simulink model "TEST1"  (R2024b)
settings: Solver=ode4  StartTime=0.0  StopTime=100  FixedStep=0.01  RelTol=1e-3
libraries: slpidlib x1, simulink x1
settings Model: LastModifiedBy=Arshaan Parwez

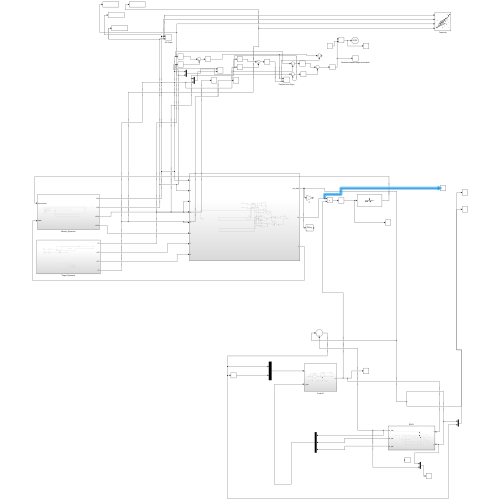
[thumbnail: Simulink's stored preview of the top-level diagram]
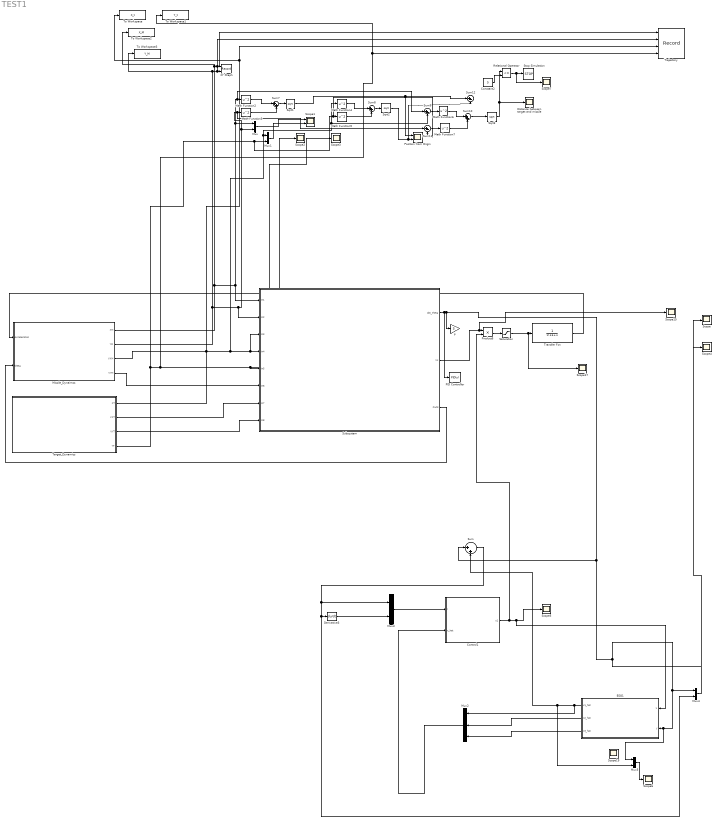
== system TEST1 ==
  Constant2 : Constant  Value=5
  Control1 : Subsystem
  Derivative3 : Derivative
  Distance between target and missile : Scope
  ESO1 : Subsystem
  Math Function{2..7} (6 alike) : Math  Operator=square
  Missile_Dynaimcs : Subsystem
  Mux{,1,3..5} (5 alike) : Mux  Inputs=2
  Mux2 : Mux  Inputs=3
  P : Gain  Gain=3
  PID Controller : slpidlib/PID Controller  Controller=PID  Form=Parallel  TimeDomain=Continuous-time  UseExternalTs=off  SampleTime=-1  IntegratorMethod=Forward Euler  FilterMethod=Forward Euler  ControllerParametersSource=internal  P=3  I=2  UseKiTs=off  D=1.5  UseExternalDerivativeSource=off  N=100  UseFilter=on  TunerSelectOption=Transfer Function Based (PID Tuner App)  InitialConditionSource=internal  InitialConditionForIntegrator=0  InitialConditionForFilter=0  DifferentiatorICPrevScaledInput=0  ExternalReset=none  TrackingMode=off  Kt=1  LimitOutput=off  SatLimitsSource=internal  UpperSaturationLimit=inf  LowerSaturationLimit=-inf  LinearizeAsGain=on  AntiWindupMode=none  Kb=1  LimitIntegrator=off  UpperIntegratorSaturationLimit=inf  LowerIntegratorSaturationLimit=-inf  POutMin=[]  POutMax=[]  IOutMin=[]  IOutMax=[]  DOutMin=[]  DOutMax=[]  NOutMin=[]  NOutMax=[]  SumOutMin=[]  SumOutMax=[]  SaturationOutMin=[]  SaturationOutMax=[]  PParamMin=[]  PParamMax=[]  IParamMin=[]  IParamMax=[]  DParamMin=[]  DParamMax=[]  NParamMin=[]  NParamMax=[]  KbParamMin=[]  KbParamMax=[]  KtParamMin=[]  KtParamMax=[]  KbOutMin=[]  KbOutMax=[]  KtOutMin=[]  KtOutMax=[]  IntegratorOutMin=[]  IntegratorOutMax=[]  FilterOutMin=[]  FilterOutMax=[]  SumI1OutMin=[]  SumI1OutMax=[]  SumI2OutMin=[]  SumI2OutMax=[]  SumI3OutMin=[]  SumI3OutMax=[]  SumI4OutMin=[]  SumI4OutMax=[]  SumDOutMin=[]  SumDOutMax=[]  DifferentiatorOutMin=[]  DifferentiatorOutMax=[]  FilterDiffOutCoefMin=[]  FilterDiffOutCoefMax=[]  ReciprocalOutMin=[]  ReciprocalOutMax=[]  SumDenOutMin=[]  SumDenOutMax=[]  SumNumOutMin=[]  SumNumOutMax=[]  DivideOutMin=[]  DivideOutMax=[]  UdiffTsProdOutMin=[]  UdiffTsProdOutMax=[]  NTsProdOutMin=[]  NTsProdOutMax=[]  UintegralTsProdOutMin=[]  UintegralTsProdOutMax=[]  UngainTsProdOutMin=[]  UngainTsProdOutMax=[]  ClampingZeroOutDataTypeStr=Inherit: Inherit via back propagation  ClampingZeroOutMin=[]  ClampingZeroOutMax=[]  FilterDenConstantOutDataTypeStr=Inherit: Inherit via back propagation  FilterDenConstantOutMin=[]  FilterDenConstantOutMax=[]  PCopyOutDataTypeStr=Inherit: Inherit via back propagation  PCopyOutMin=[]  PCopyOutMax=[]  NCopyOutDataTypeStr=Inherit: Inherit via back propagation  NCopyOutMin=[]  NCopyOutMax=[]  IntegratorContinuousStateAttributes=''  IntegratorStateMustResolveToSignalObject=off  IntegratorRTWStateStorageClass=Auto  FilterContinuousStateAttributes=''  FilterStateMustResolveToSignalObject=off  FilterRTWStateStorageClass=Auto  ParallelPVariant=InternalParameters  IdealPVariant=Disabled  IVariant=InternalParameters  DVariant=InternalParameters  IntegratorVariant=Continuous  SatVariant=Disabled  AWVariant=Passthrough  PCopyVariant=Disabled  TRVariant=Disabled  FdbkBlocksVariant=Forward  IdealPFdbkVariant=Disabled  SatFdbkVariant=Disabled  DerivativeFilterVariant=ContFilter  NVariant=InternalParameters  NCopyVariant=Disabled  FilterICVariant=InternalICsFilter  IntegratorICVariant=InternalICs  ExternalResetVariant=Disabled  TRSumVariant=Passthrough  SumFdbkVariant=Disabled  SumVariant=Sum_PID  TsampFilterVariant=InternalTs  TsampNgainVariant=Passthrough  TsampIntegralVariant=Disabled_SignalSpec  ExternalSaturationOutDataTypeStr=Inherit: Same as second input  DerivativeSourceVariant=ErrorSignal  PreIntVariant=InternalPreInt
  Position from Origin : Scope  NumInputPorts=2
  Product6 : Product
  Relational Operator : RelationalOperator  Operator=<=  OutDataTypeStr=boolean  RndMeth=Simplest  InputSameDT=off
  Saturation : Saturate  UpperLimit=50  LowerLimit=-50
  Scope{,2..7,15,17,19} (10 alike) : Scope
  Scope1 : Scope  NumInputPorts=2
  Sqrt1 : Sqrt
  Sqrt2 : Sqrt
  Sqrt3 : Sqrt
  Stop Simulation : Stop
  Subsystem : Subsystem
  Sum{,7..8,10} (4 alike) : Sum  Inputs=|++
  Sum11 : Sum  Inputs=|+-
  Sum12 : Sum  Inputs=|+-
  Sum9 : Sum  Inputs=|+-
  Target_Dynamics : Subsystem
  To Workspace : ToWorkspace  VariableName=X_t  SaveFormat=Timeseries  SampleTime=-1
  To Workspace1 : ToWorkspace  VariableName=Y_t  SaveFormat=Timeseries  SampleTime=-1
  To Workspace2 : ToWorkspace  VariableName=X_M  SaveFormat=Timeseries  SampleTime=-1
  To Workspace3 : ToWorkspace  VariableName=Y_M  SaveFormat=Timeseries  SampleTime=-1
  Trajectory : Record  FileSettingsInternal="{\"entries\":[{\"content\":{\"excelSettings\":{\"content\":{},\"type\":\"Streamout.ExcelSettings\"}},\"type\":\"Streamout.FileSettingStorage\",\"uuid\":\"\"}],\"packageUris\":[\"http:\\/\\/schema.mathworks.com\\/mf0\\/streamout_blocks\\/R2020a\"],\"version\":\"1.0\"}"  Layout=[1 1]  SignalsInternal="{\"entries\":[{\"content\":{\"signals\":[{\"content\":{\"blockPath\":[],\"dimensions\":[1],\"domain\":\"\",\"lineColor\":\"#fe330a\",\"lineWidth\":2,\"plots\":[ 1 ],\"port\":1,\"sid\":[\"\"],\"signalID\":1,\"signalName\":\"Missile_Dynaimcs:1\"},\"type\":\"RecordBlkView.Signal\",\"uuid\":\"\"},{\"content\":{\"blockPath\":[],\"dimensions\":[1],\"domain\":\"\",\"lineColor\":\"#d95319\",\"lineWidth\":2,\"plots\":[ 1 ],\"port\":2,\"sid\":[\"\"],\"signalID\":2,\"signalName\":\"Missile_Dynaimcs:2\"},\"type\":\"RecordBlkView.Signal\",\"uuid\":\"\"},{\"content\":{\"blockPath\":[],\"dimensions\":[1],\"domain\":\"\",\"lineColor\":\"#0072bd\",\"lineWidth\":2,\"plots\":[ 1 ],\"port\":3,\"sid\":[\"\"],\"signalID\":3,\"signalName\":\"Target_Dynamics:1\"},\"type\":\"RecordBlkView.Signal\",\"uuid\":\"\"},{\"content\":{\"blockPath\":[],\"dimensions\":[1],\"domain\":\"\",\"lineColor\":\"#0072bd\",\"lineWidth\":2,\"plots\":[ 1 ],\"port\":4,\"sid\":[\"\"],\"signalID\":4,\"signalName\":\"Target_Dynamics:4\"},\"type\":\"RecordBlkView.Signal\",\"uuid\":\"\"}]},\"type\":\"RecordBlkView.InputSignals\",\"uuid\":\"\"}],\"packageUris\":[\"http:\\/\\/schema.mathworks.com\\/mf0\\/streamout_blocks\\/R2020a\"],\"version\":\"1.0\"}"  VisualizationBindings="{\"xyplotplugin\":{\"info\":[{\"series\":[{\"bindingParametersList\":[{\"parameter\":\"X-Axis\",\"signalID\":1,\"signalName\":\"Missile_Dynaimcs:1\"},{\"parameter\":\"Y-Axis\",\"signalID\":2,\"signalName\":\"Missile_Dynaimcs:2\"}],\"seriesID\":0},{\"bindingParametersList\":[{\"parameter\":\"X-Axis\",\"signalID\":3,\"signalName\":\"Target_Dynamics:1\"},{\"parameter\":\"Y-Axis\",\"signalID\":4,\"signalName\":\"Target_Dynamics:4\"}],\"seriesID\":1}],\"subplotID\":1}]}}"  CompatibilityTag=XY
  Transfer Fcn : TransferFcn  Denominator=[0.1 1]
  XY Graph : Record  FileSettingsInternal="{\"entries\":[{\"content\":{\"excelSettings\":{\"content\":{},\"type\":\"Streamout.ExcelSettings\"}},\"type\":\"Streamout.FileSettingStorage\",\"uuid\":\"\"}],\"packageUris\":[\"http:\\/\\/schema.mathworks.com\\/mf0\\/streamout_blocks\\/R2020a\"],\"version\":\"1.0\"}"  Layout=[1 1]  SignalsInternal="{\"entries\":[{\"content\":{\"signals\":[{\"content\":{\"blockPath\":[],\"dimensions\":[1],\"domain\":\"\",\"lineColor\":\"#64d413\",\"lineWidth\":2,\"port\":1,\"sid\":[\"\"],\"signalID\":1,\"signalName\":\"Missile_Dynaimcs:1\"},\"type\":\"RecordBlkView.Signal\",\"uuid\":\"\"},{\"content\":{\"blockPath\":[],\"dimensions\":[1],\"domain\":\"\",\"lineColor\":\"#ff13a6\",\"lineWidth\":2,\"port\":2,\"sid\":[\"\"],\"signalID\":2,\"signalName\":\"Missile_Dynaimcs:2\"},\"type\":\"RecordBlkView.Signal\",\"uuid\":\"\"}]},\"type\":\"RecordBlkView.InputSignals\",\"uuid\":\"\"}],\"packageUris\":[\"http:\\/\\/schema.mathworks.com\\/mf0\\/streamout_blocks\\/R2020a\"],\"version\":\"1.0\"}"  VisualizationBindings="{\"xyplotplugin\":{\"info\":[{\"series\":[],\"subplotID\":1}]}}"  CompatibilityTag=XY
  wires:
  Transfer Fcn/1 -> Missile_Dynaimcs/1(Acceleration)
  Mux/1 -> Scope1/1
  Mux1/1 -> Scope1/2
  Math Function2/1 -> Sum7/1
  Math Function3/1 -> Sum7/2
  Sum7/1 -> Sqrt1/1
  Math Function4/1 -> Sum8/1
  Sum8/1 -> Sqrt2/1
  Math Function5/1 -> Sum8/2
  Sqrt1/1 -> Sum12/1, Position from Origin/1
  Sqrt2/1 -> Sum12/2, Position from Origin/2
  Relational Operator/1 -> Scope7/1, Stop Simulation/1
  Sum9/1 -> Math Function6/1
  Sum11/1 -> Math Function7/1
  Math Function6/1 -> Sum10/1
  Math Function7/1 -> Sum10/2
  Sum10/1 -> Sqrt3/1
  Constant2/1 -> Relational Operator/2
  Target_Dynamics/1(XT) -> To Workspace/1, Trajectory/3, Math Function4/1, Sum9/2, Mux1/1, Scope2/1, Subsystem/3(In3)
  Target_Dynamics/4(YT) -> Sum11/2, Math Function5/1, Mux1/2, To Workspace1/1, Trajectory/4, Scope3/1, Subsystem/5(In5)
  Missile_Dynaimcs/1(XM) -> To Workspace2/1, Trajectory/1, XY Graph/1, Subsystem/1(In1), Sum9/1, Math Function2/1, Mux/1
  Missile_Dynaimcs/2(YM) -> To Workspace3/1, Trajectory/2, XY Graph/2, Subsystem/2(In2), Sum11/1, Math Function3/1, Mux/2
  Missile_Dynaimcs/3(VXM) -> Subsystem/4(In4)
  Missile_Dynaimcs/4(VYM) -> Subsystem/6(In6)
  Target_Dynamics/2(VXT) -> Subsystem/7(In7)
  Target_Dynamics/3(VYT) -> Subsystem/8(In8)
  Subsystem/3(Out3) -> Missile_Dynaimcs/2(theta)
  Sqrt3/1 -> Distance between target and missile/1, Relational Operator/1
  Derivative3/1 -> Mux3/2
  Mux3/1 -> Control1/1(r)
  Sum/1 -> Mux4/2, Derivative3/1, Mux3/1
  ESO1/1(x1_hat) -> Mux2/1, Sum/2, Mux5/2
  Mux2/1 -> Control1/2(x_hat)
  Mux4/1 -> Scope4/1
  Mux5/1 -> Scope6/1
  Subsystem/1(dot_theta) -> PID Controller/1, P/1, Sum/1, Mux4/1, ESO1/2(y), Mux5/1, Scope/1
  Control1/1(u1) -> Product6/2, ESO1/1(u), Scope5/1
  Subsystem/2(Vc) -> Scope15/1, Product6/1
  ESO1/2(x2_hat) -> Mux2/2
  ESO1/3(x3_hat) -> Mux2/3
  Product6/1 -> Saturation/1
  Saturation/1 -> Scope17/1, Transfer Fcn/1

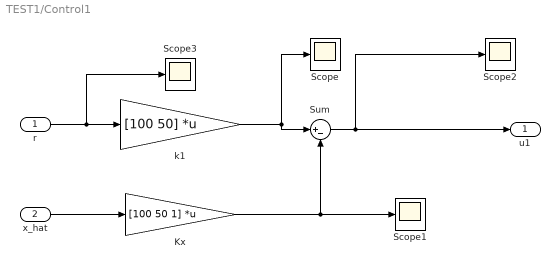
== system TEST1/Control1 ==
  r : Inport
  x_hat : Inport  Port=2
  Kx : Gain  Gain=[100 50 1]  Multiplication=Matrix(K*u)
  Scope{,1..3} (4 alike) : Scope
  Sum : Sum  Inputs=|+-
  k1 : Gain  Gain=[100 50]  Multiplication=Matrix(K*u)
  u1 : Outport
  wires:
  Sum/1 -> u1/1, Scope2/1
  Kx/1 -> Scope1/1, Sum/2
  k1/1 -> Sum/1, Scope/1
  x_hat/1 -> Kx/1
  r/1 -> Scope3/1, k1/1

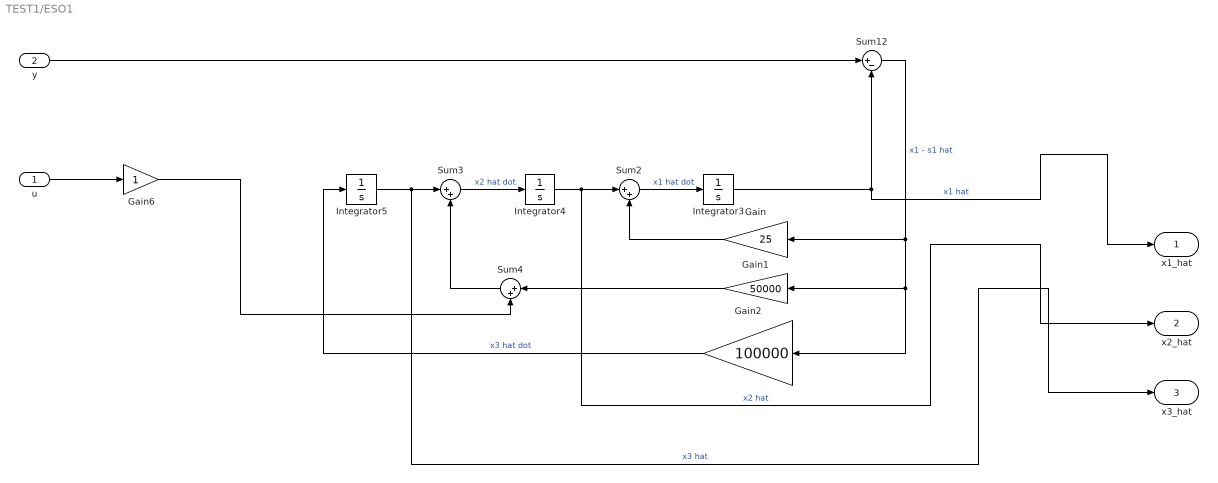
== system TEST1/ESO1 ==
  u : Inport
  y : Inport  Port=2
  Gain : Gain  Gain=25
  Gain1 : Gain  Gain=50000
  Gain2 : Gain  Gain=100000
  Gain6 : Gain
  Integrator3 : Integrator
  Integrator4 : Integrator
  Integrator5 : Integrator
  Sum12 : Sum  Inputs=|+-
  Sum2 : Sum  Inputs=|++
  Sum3 : Sum  Inputs=|++
  Sum4 : Sum  Inputs=|++
  x1_hat : Outport
  x2_hat : Outport  Port=2
  x3_hat : Outport  Port=3
  wires:
  Gain1/1 -> Sum4/1
  Sum12/1 -> Gain/1, Gain1/1, Gain2/1  "x1 - s1 hat"
  Sum4/1 -> Sum3/2
  Integrator4/1 -> x2_hat/1, Sum2/1  "x2 hat"
  Integrator3/1 -> x1_hat/1, Sum12/2  "x1 hat"
  Gain2/1 -> Integrator5/1  "x3 hat dot"
  y/1 -> Sum12/1
  u/1 -> Gain6/1
  Sum3/1 -> Integrator4/1  "x2 hat dot"
  Gain6/1 -> Sum4/2
  Gain/1 -> Sum2/2
  Integrator5/1 -> Sum3/1, x3_hat/1  "x3 hat"
  Sum2/1 -> Integrator3/1  "x1 hat dot"

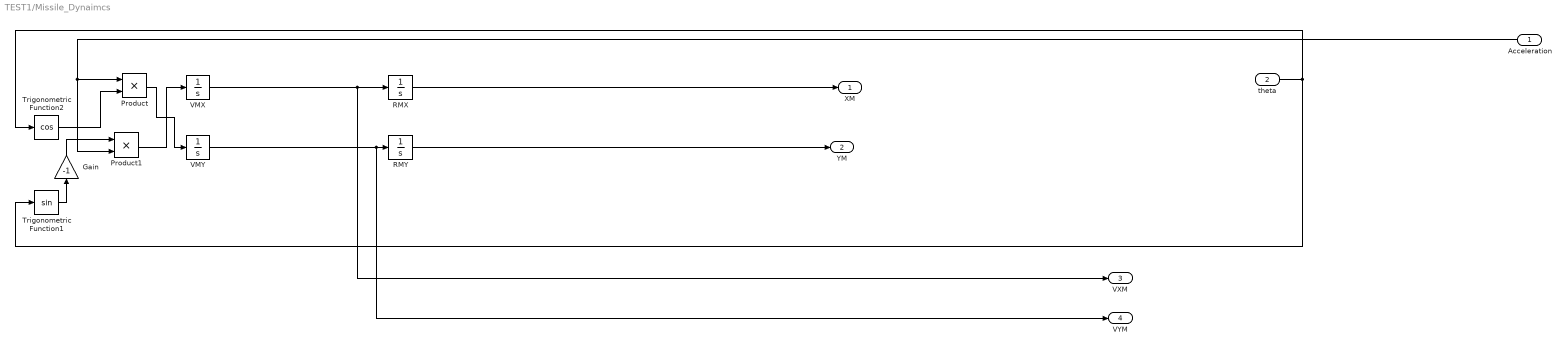
== system TEST1/Missile_Dynaimcs ==
  Acceleration : Inport
  theta : Inport  Port=2
  Gain : Gain  Gain=-1
  Product : Product
  Product1 : Product
  RMX : Integrator
  RMY : Integrator  InitialCondition=3000
  Trigonometric Function1 : Trigonometry
  Trigonometric Function2 : Trigonometry  Operator=cos
  VMX : Integrator  InitialCondition=600
  VMY : Integrator  InitialCondition=100
  XM : Outport
  YM : Outport  Port=2
  VXM : Outport  Port=3
  VYM : Outport  Port=4
  wires:
  Trigonometric Function1/1 -> Gain/1
  VMX/1 -> VXM/1, RMX/1
  theta/1 -> Trigonometric Function1/1, Trigonometric Function2/1
  Trigonometric Function2/1 -> Product/2
  RMX/1 -> XM/1
  Acceleration/1 -> Product1/2, Product/1
  Product/1 -> VMY/1
  Product1/1 -> VMX/1
  VMY/1 -> VYM/1, RMY/1
  Gain/1 -> Product1/1
  RMY/1 -> YM/1

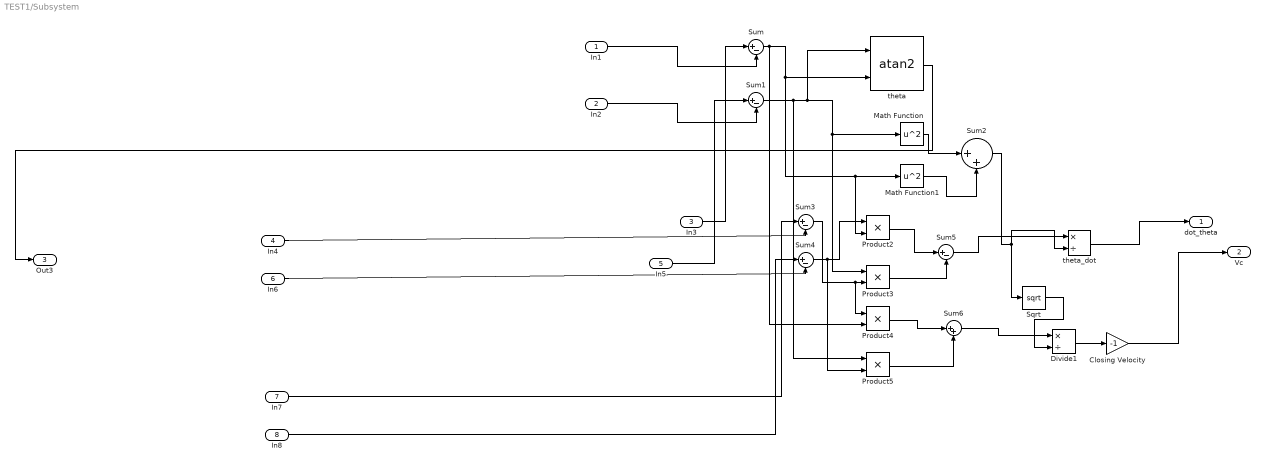
== system TEST1/Subsystem ==
  In1 : Inport
  In2 : Inport  Port=2
  In3 : Inport  Port=3
  In4 : Inport  Port=4
  In5 : Inport  Port=5
  In6 : Inport  Port=6
  In7 : Inport  Port=7
  In8 : Inport  Port=8
  Closing Velocity : Gain  Gain=-1
  Divide1 : Product  Inputs=*/
  Math Function : Math  Operator=square
  Math Function1 : Math  Operator=square
  Product{2..5} (4 alike) : Product
  Sqrt : Sqrt
  Sum{,1,3..5} (5 alike) : Sum  Inputs=|+-
  Sum2 : Sum  Inputs=|++
  Sum6 : Sum  Inputs=|++
  theta : Trigonometry  Operator=atan2
  theta_dot : Product  Inputs=*/
  dot_theta : Outport
  Vc : Outport  Port=2
  Out3 : Outport  Port=3
  wires:
  Math Function/1 -> Sum2/1
  Sum2/1 -> Sqrt/1, theta_dot/2
  Sum3/1 -> Product4/1, Product3/2
  Sum/1 -> Product4/2, Product2/2, Math Function1/1, theta/2
  Product4/1 -> Sum6/1
  Product2/1 -> Sum5/1
  Sum6/1 -> Divide1/1
  Math Function1/1 -> Sum2/2
  Sum4/1 -> Product5/2, Product2/1
  Sqrt/1 -> Divide1/2
  Divide1/1 -> Closing Velocity/1
  Product5/1 -> Sum6/2
  In3/1 -> Sum/1
  In7/1 -> Sum3/1
  Sum1/1 -> Product5/1, Product3/1, Math Function/1, theta/1
  theta_dot/1 -> dot_theta/1
  In8/1 -> Sum4/1
  In1/1 -> Sum/2
  theta/1 -> Out3/1
  Closing Velocity/1 -> Vc/1
  In5/1 -> Sum1/1
  In4/1 -> Sum3/2
  Product3/1 -> Sum5/2
  Sum5/1 -> theta_dot/1
  In2/1 -> Sum1/2
  In6/1 -> Sum4/2

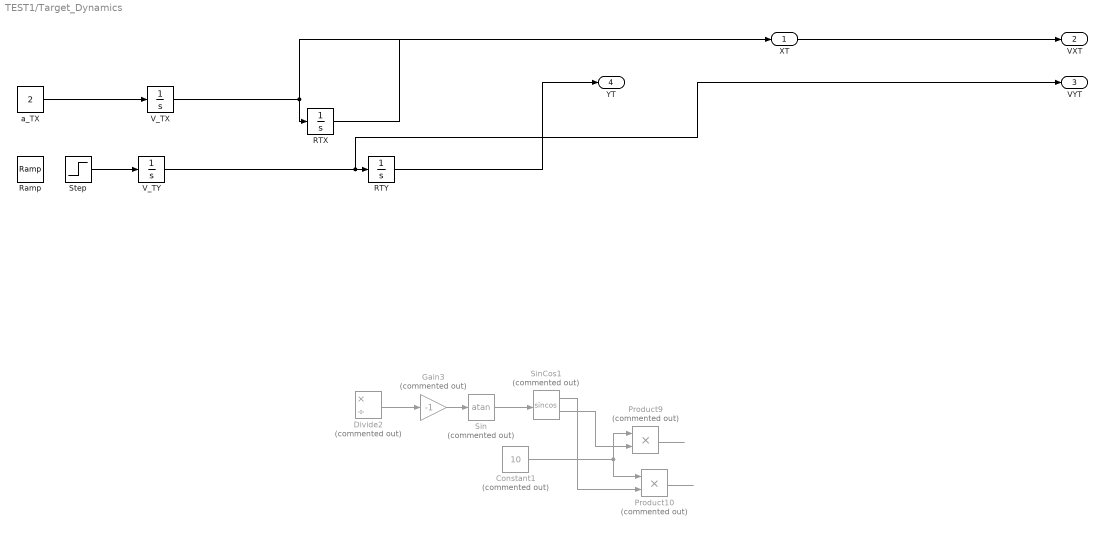
== system TEST1/Target_Dynamics ==
  Constant1 : Constant  Commented=on  Value=10
  Divide2 : Product  Commented=on  Inputs=*/
  Gain3 : Gain  Commented=on  Gain=-1
  Product10 : Product  Commented=on
  Product9 : Product  Commented=on
  RTX : Integrator  InitialCondition=11000
  RTY : Integrator  InitialCondition=3000
  Ramp : simulink/Sources/Ramp  slope=-0.75  start=0  InitialOutput=0
  Sin : Trigonometry  Commented=on  Operator=atan
  SinCos1 : Trigonometry  Commented=on  Operator=sincos
  Step : Step  Time=15  Before=-4  After=-10  SampleTime=0
  V_TX : Integrator  InitialCondition=150
  V_TY : Integrator  InitialCondition=100
  a_TX : Constant  Value=2
  XT : Outport
  VXT : Outport  Port=2
  VYT : Outport  Port=3
  YT : Outport  Port=4
  wires:
  SinCos1/1 -> Product10/2
  Product9/1 -> ?
  SinCos1/2 -> Product9/2
  Divide2/1 -> Gain3/1
  Constant1/1 -> Product10/1, Product9/1
  Gain3/1 -> Sin/1
  Sin/1 -> SinCos1/1
  a_TX/1 -> V_TX/1
  RTX/1 -> XT/1
  Product10/1 -> ?
  RTY/1 -> YT/1
  V_TX/1 -> VXT/1, RTX/1
  V_TY/1 -> VYT/1, RTY/1
  Step/1 -> V_TY/1
